simulink model "PID"  (R2020b)
settings: Solver=VariableStepAuto  StartTime=0.0  StopTime=10.0  RelTol=1e-3
undefined symbols (not defined in the file): National_Instruments, PCI
libraries: sldrtlib x2, pid_lib x1, simulink x1
settings Model: Creator=diosdado  LastModifiedBy=diosdado

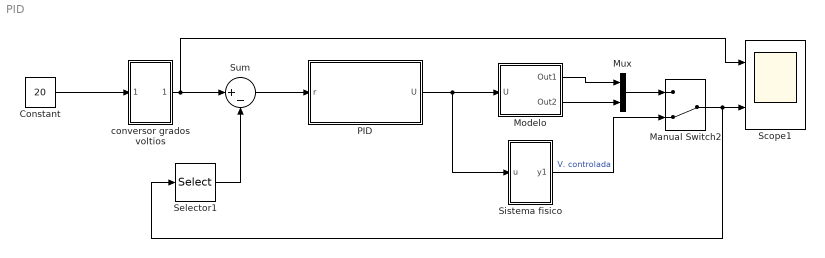
== system PID ==
  Constant : Constant  Value=20
  Manual Switch2 : ManualSwitch  CurrentSetting=0
  "Modelo " : Subsystem
  Mux : Mux  Inputs=2
  PID : Subsystem
  Scope1 : Scope  NumInputPorts=2
  Selector1 : Selector  InputPortWidth=2  IndexOptions=Index vector (dialog)  Indices=[1]  OutputSizes=1
  Sistema fisico : Subsystem
  Sum : Sum  Inputs=|+-
  "conversor grados voltios " : Subsystem  mask{a=4.95, b=0.869}
  wires:
  Constant/1 -> "conversor grados voltios "/1(In1)
  "conversor grados voltios "/1(Out1) -> Scope1/1, Sum/1
  Selector1/1 -> Sum/2
  Sum/1 -> PID/1(r)
  PID/1(U) -> Sistema fisico/1(u), "Modelo "/1(U)
  "Modelo "/2(Out2) -> Mux/2
  "Modelo "/1(Out1) -> Mux/1
  Mux/1 -> Manual Switch2/1
  Sistema fisico/1(y1) -> Manual Switch2/2  "V. controlada"
  Manual Switch2/1 -> Selector1/1, Scope1/2

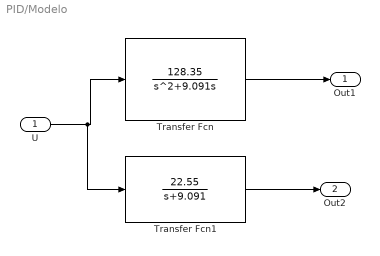
== system PID/Modelo  ==
  U : Inport
  Transfer Fcn : TransferFcn  Numerator=[128.35]  Denominator=[1 9.091 0]
  Transfer Fcn1 : TransferFcn  Numerator=[22.55]  Denominator=[1 9.091]
  Out1 : Outport
  Out2 : Outport  Port=2
  wires:
  U/1 -> Transfer Fcn1/1, Transfer Fcn/1
  Transfer Fcn/1 -> Out1/1
  Transfer Fcn1/1 -> Out2/1

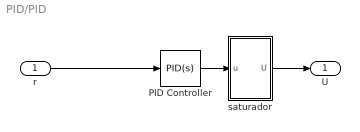
== system PID/PID ==
  r : Inport
  PID Controller : pid_lib/PID Controller  Controller=PID  Form=Parallel  TimeDomain=Continuous-time  UseExternalTs=off  SampleTime=-1  IntegratorMethod=Forward Euler  FilterMethod=Forward Euler  ControllerParametersSource=internal  P=1.17  I=1.96  D=0.118  UseFilter=on  N=100  TunerSelectOption=Transfer Function Based (PID Tuner App)  InitialConditionSource=internal  InitialConditionForIntegrator=0  InitialConditionForFilter=0  DifferentiatorICPrevScaledInput=0  ExternalReset=none  TrackingMode=off  Kt=1  LimitOutput=off  SatLimitsSource=internal  UpperSaturationLimit=inf  LowerSaturationLimit=-inf  LinearizeAsGain=on  AntiWindupMode=none  Kb=1  POutMin=[]  POutMax=[]  IOutMin=[]  IOutMax=[]  DOutMin=[]  DOutMax=[]  NOutMin=[]  NOutMax=[]  SumOutMin=[]  SumOutMax=[]  SaturationOutMin=[]  SaturationOutMax=[]  PParamMin=[]  PParamMax=[]  IParamMin=[]  IParamMax=[]  DParamMin=[]  DParamMax=[]  NParamMin=[]  NParamMax=[]  KbParamMin=[]  KbParamMax=[]  KtParamMin=[]  KtParamMax=[]  KbOutMin=[]  KbOutMax=[]  KtOutMin=[]  KtOutMax=[]  IntegratorOutMin=[]  IntegratorOutMax=[]  FilterOutMin=[]  FilterOutMax=[]  SumI1OutMin=[]  SumI1OutMax=[]  SumI2OutMin=[]  SumI2OutMax=[]  SumI3OutMin=[]  SumI3OutMax=[]  SumI4OutMin=[]  SumI4OutMax=[]  SumDOutMin=[]  SumDOutMax=[]  DifferentiatorOutMin=[]  DifferentiatorOutMax=[]  FilterDiffOutCoefMin=[]  FilterDiffOutCoefMax=[]  ReciprocalOutMin=[]  ReciprocalOutMax=[]  SumDenOutMin=[]  SumDenOutMax=[]  SumNumOutMin=[]  SumNumOutMax=[]  DivideOutMin=[]  DivideOutMax=[]  UdiffTsProdOutMin=[]  UdiffTsProdOutMax=[]  NTsProdOutMin=[]  NTsProdOutMax=[]  UintegralTsProdOutMin=[]  UintegralTsProdOutMax=[]  UngainTsProdOutMin=[]  UngainTsProdOutMax=[]  IntegratorContinuousStateAttributes=''  IntegratorStateMustResolveToSignalObject=off  IntegratorRTWStateStorageClass=Auto  FilterContinuousStateAttributes=''  FilterStateMustResolveToSignalObject=off  FilterRTWStateStorageClass=Auto  ParallelPVariant=InternalParameters  IdealPVariant=Disabled  IVariant=InternalParameters  DVariant=InternalParameters  IntegratorVariant=Continuous  SatVariant=Disabled  AWVariant=Passthrough  PCopyVariant=Disabled  TRVariant=Disabled  FdbkBlocksVariant=Forward  IdealPFdbkVariant=Disabled  SatFdbkVariant=Disabled  DerivativeFilterVariant=ContFilter  NVariant=InternalParameters  NCopyVariant=Disabled  FilterICVariant=InternalICsFilter  IntegratorICVariant=InternalICs  ExternalResetVariant=Disabled  TRSumVariant=Passthrough  SumFdbkVariant=Disabled  SumVariant=Sum_PID  TsampFilterVariant=InternalTs  TsampNgainVariant=Passthrough  TsampIntegralVariant=Passthrough  ExternalSaturationOutDataTypeStr=Inherit: Same as second input
  saturador : Subsystem
  U : Outport
  wires:
  PID Controller/1 -> saturador/1(u)
  r/1 -> PID Controller/1
  saturador/1(U) -> U/1

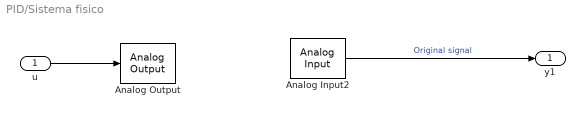
== system PID/Sistema fisico ==
  u : Inport
  Analog Input2 : sldrtlib/Analog Input  SampleTime=0.001  MaxMissedTicks=10  ShowMissedTicks=off  YieldWhenWaiting=off  DrvName=National_Instruments/PCI-6014  DrvAddress=4294967295  DrvOptions=[2 0 0 0 0 0]  Channels=[1,2]  RangeMode=1  VoltRange=1  DataType=1
      settings: AttributesFormatString=National Instruments\nPCI-6014 [auto]
  Analog Output : sldrtlib/Analog Output  SampleTime=0.001  MaxMissedTicks=10  ShowMissedTicks=off  YieldWhenWaiting=off  DrvName=National_Instruments/PCI-6014  DrvAddress=4294967295  DrvOptions=[2 0 0 0 0 0]  Channels=1  RangeMode=1  VoltRange=1  InitialValue=[]  FinalValue=[]
      settings: AttributesFormatString=National Instruments\nPCI-6014 [auto]
  y1 : Outport
  wires:
  u/1 -> Analog Output/1
  Analog Input2/1 -> y1/1  "Original signal"

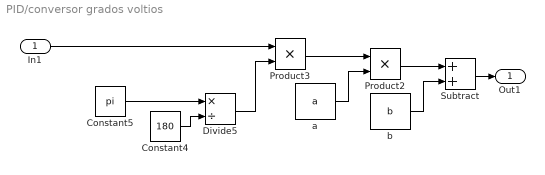
== system PID/conversor grados voltios  ==
  In1 : Inport
  Constant4 : Constant  Value=180
  Constant5 : Constant  Value=pi
  Divide5 : Product  Inputs=*/
  Product2 : Product
  Product3 : Product
  Subtract : Sum
  a : Constant  Value=a
  b : Constant  Value=b
  Out1 : Outport
  wires:
  b/1 -> Subtract/2
  Product3/1 -> Product2/1
  Constant4/1 -> Divide5/2
  In1/1 -> Product3/1
  Product2/1 -> Subtract/1
  a/1 -> Product2/2
  Constant5/1 -> Divide5/1
  Divide5/1 -> Product3/2
  Subtract/1 -> Out1/1

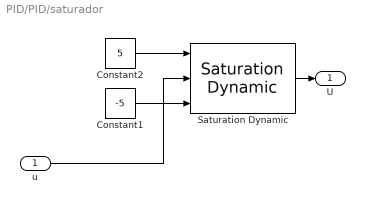
== system PID/PID/saturador ==
  u : Inport  OutDataTypeStr=double
  Constant1 : Constant  Value=-5
  Constant2 : Constant  Value=5
  Saturation Dynamic : simulink/Discontinuities/Saturation Dynamic  OutMin=-5  OutMax=5  OutDataTypeStr=Inherit: Same as second input  OutDataType=fixdt(1, 16)  OutScaling=2^-10  DoSatur=off
  U : Outport  OutDataTypeStr=double
  wires:
  u/1 -> Saturation Dynamic/2
  Constant2/1 -> Saturation Dynamic/1
  Saturation Dynamic/1 -> U/1
  Constant1/1 -> Saturation Dynamic/3
